simulink model "Model_sim"  (R2024b)
settings: Solver=VariableStepAuto  StartTime=0.0  StopTime=10000  RelTol=1e-3
values from neighbouring files (symbols this model uses):
  x0 = [r10;alfa(:,i)+r20;d_r10;d_r20;eps0]    [Model_OrbitaSateliti.m]
settings Model: Creator=mihne  LastModifiedBy=Mihnea

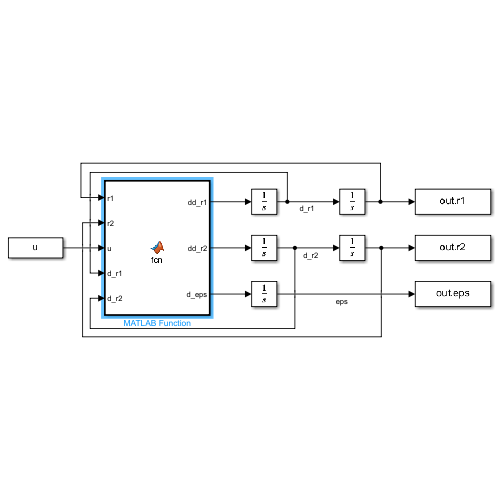
[thumbnail: Simulink's stored preview of the top-level diagram]
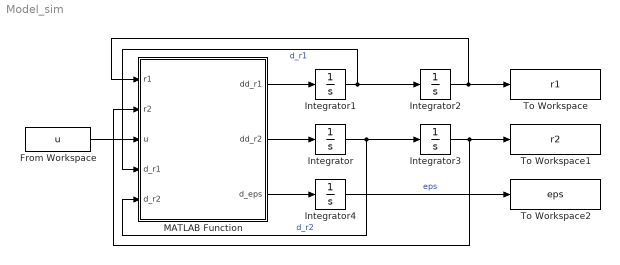
== system Model_sim ==
  From Workspace : FromWorkspace  VariableName=u
  Integrator : Integrator  InitialCondition=x0(10:12)
  Integrator1 : Integrator  InitialCondition=x0(7:9)
  Integrator2 : Integrator  InitialCondition=x0(1:3)
  Integrator3 : Integrator  InitialCondition=x0(4:6)
  Integrator4 : Integrator  InitialCondition=x0(13)
  MATLAB Function : MATLAB Function  TreatAsAtomicUnit=on
  To Workspace : ToWorkspace  VariableName=r1  SaveFormat=Timeseries  SampleTime=-1
  To Workspace1 : ToWorkspace  VariableName=r2  SaveFormat=Timeseries  SampleTime=-1
  To Workspace2 : ToWorkspace  VariableName=eps  SaveFormat=Timeseries  SampleTime=-1
  wires:
  MATLAB Function/2(dd_r2) -> Integrator/1
  MATLAB Function/1(dd_r1) -> Integrator1/1
  Integrator/1 -> Integrator3/1, MATLAB Function/5(d_r2)  "d_r2"
  Integrator1/1 -> Integrator2/1, MATLAB Function/4(d_r1)  "d_r1"
  Integrator2/1 -> To Workspace/1, MATLAB Function/1(r1)
  Integrator3/1 -> To Workspace1/1, MATLAB Function/2(r2)
  MATLAB Function/3(d_eps) -> Integrator4/1
  From Workspace/1 -> MATLAB Function/3(u)
  Integrator4/1 -> To Workspace2/1  "eps"

== matlab function Model_sim/MATLAB Function ==
  data: r1 input; r2 input; u input; d_r1 input; d_r2 input; dd_r1 output; dd_r2 output; d_eps output
function [dd_r1, dd_r2, d_eps] = fcn(r1, r2, u, d_r1, d_r2)
dd_r1=g(r1,d_r1)+u;
dd_r2=g(r2,d_r2);
d_eps=norm(r1-r2)/norm(r2);
